simulink model "ADC2019"  (R2019b)
settings: Solver=VariableStepAuto  StartTime=0.0  StopTime=1  RelTol=1e-3
values from neighbouring files (symbols this model uses):
  Cf = minimum_cap    [SignalProcessing_SAR.m]    (also in simVariables.mat = 1.995e-15)
  clk_period = 1/clk_freq    [SignalProcessing_SAR.m]    (also in simVariables.mat = 5.92094282336e-05)
  comparator_high_offset = 8e-4    (= 0.0008)    [SignalProcessing_SAR.m]    (also in simVariables.mat)
  comparator_low_offset = 8e-4    (= 0.0008)    [SignalProcessing_SAR.m]    (also in simVariables.mat)
  comparator_noise_on = non_idealities_on    (= 1)    [SignalProcessing_SAR.m]    (also in simVariables.mat)
  comparator_noise_rms = 1*k*T* 2/3 / minimum_cap    [SignalProcessing_SAR.m]    (also in simVariables.mat = 1.35181292017e-06)
  comparator_offset_on = non_idealities_on    (= 1)    [SignalProcessing_SAR.m]    (also in simVariables.mat)
  k = 1.38064852e-23    [SignalProcessing_SAR.m]    (also in simVariables.mat)
  LNA_bandwidth = 30*input_BW    (= 7680)    [SignalProcessing_SAR.m]    (also in simVariables.mat)
  LNA_gain = 100    [SignalProcessing_SAR.m]    (also in simVariables.mat)
  LNA_input_referred_noise = min([LNA_input_referred_noise_1,LNA_input_referred_noise_2,LNA_input_referred_noise_3])    [SignalProcessing_SAR.m]    (also in simVariables.mat = 3.60843918244e-05)
  LNA_noise_on = non_idealities_on    (= 1)    [SignalProcessing_SAR.m]    (also in simVariables.mat)
  LNA_SR = I_LNA/(minimum_cap)    [SignalProcessing_SAR.m]    (also in simVariables.mat = 4429889.66082)
  number_of_bits = nb_bits    [SignalProcessing_SAR.m]    (also in simVariables.mat = 4)
  sample_time_jitter = 16e-12    (= 1.6e-11)    [SignalProcessing_SAR.m]    (also in simVariables.mat)
  sampling_gain = Cs/Cf    [SignalProcessing_SAR.m]    (also in simVariables.mat = 10)
  sampling_jitter_on = non_idealities_on    (= 1)    [SignalProcessing_SAR.m]    (also in simVariables.mat)
  switch_noise_on = non_idealities_on    (= 1)    [SignalProcessing_SAR.m]    (also in simVariables.mat)
  switching_noise = k*T/Cf    [SignalProcessing_SAR.m]    (also in simVariables.mat = 2.02771938025e-06)
  T = 293    [SignalProcessing_SAR.m]    (also in simVariables.mat)
  Vref = 2    [SignalProcessing_SAR.m]    (also in simVariables.mat)
undefined symbols (not defined in the file or in its folder): sim_number
libraries: dspsigops x2, spsFirstOrderFilterLib x1, simulink x1, simulink_extras x1, dspsrcs4 x1
settings Model: SnapshotInterval=1  Creator=mac  LastModifiedBy=mac
settings DataIOCC: SaveFormat=Structure  OutputOption=SpecifiedOutputTimes  OutputTimes=0:(clk_period*(number_of_bits+1)): length(ADC_input)*(number_of_bits+1)*clk_period
settings DebuggingCC: UnderSpecifiedDimensionMsg=warning

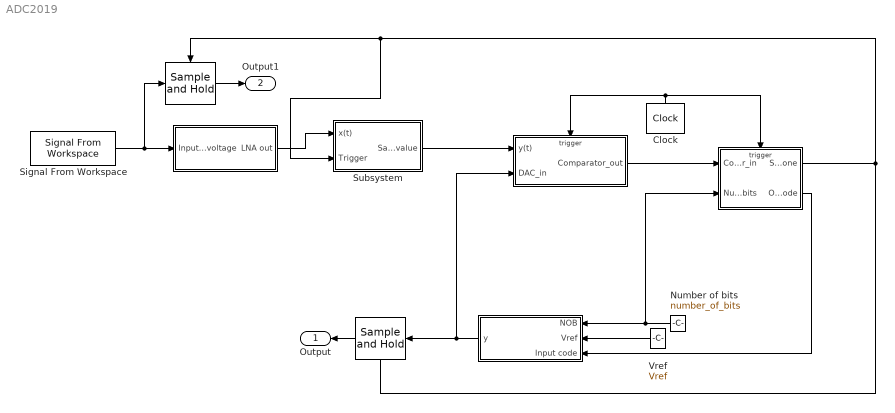
== system ADC2019 ==
  " " : Subsystem
      mask Display: text(.5, .5, 'LNA', 'horizontalAlignment', 'center', 'verticalAlignment', 'middle')
  "  " : Subsystem  TreatAsAtomicUnit=on
      mask Display: text(.5, .5, 'Comparator', 'horizontalAlignment', 'center', 'verticalAlignment', 'middle')
  "    " : Subsystem  TreatAsAtomicUnit=on
      mask Display: text(.5, .5, 'SAR', 'horizontalAlignment', 'center', 'verticalAlignment', 'middle')
  "       " : Subsystem  TreatAsAtomicUnit=on
      mask Display: text(.5, .5, 'DAC', 'horizontalAlignment', 'center', 'verticalAlignment', 'middle')
  "          " : dspsigops/Sample and Hold  trig=Rising edge  initCond=0  latchinput=off
  "           " : dspsigops/Sample and Hold  trig=Rising edge  initCond=0  latchinput=off
  Clock : simulink_extras/Flip Flops/Clock  period=clk_period
  Number of bits : Constant  Value=number_of_bits
  Signal From Workspace : dspsrcs4/Signal From Workspace  X=ADC_input  Ts=clk_period*(number_of_bits+1)  nsamps=1  OutputAfterFinalValue=Setting to zero  ignoreOrWarnInputAndFrameLengths=off  OutputFrames=off
  Subsystem : Subsystem
      mask Display: text(.5, .5, 'Sample & hold', 'horizontalAlignment', 'center', 'verticalAlignment', 'middle')
  Vref : Constant  Value=Vref
  Output : Outport
  Output1 : Outport  Port=2
  wires:
  Vref/1 -> "       "/2(Vref)
  "    "/2(Output_code) -> "       "/3(Input code)
  Clock/1 -> "    "/Trigger, "  "/Trigger
  "       "/1(y) -> "           "/1, "  "/2(DAC_in)
  "  "/1(Comparator_out) -> "    "/1(Comparator_in)
  "           "/1 -> Output/1
  " "/1(LNA out) -> Subsystem/1(x(t))
  Subsystem/1(Sampled value) -> "  "/1(y(t))
  Number of bits/1 -> "    "/2(Number of bits), "       "/1(NOB)
  "    "/1(SAR_done) -> "           "/Trigger, Subsystem/2(Trigger), "          "/Trigger
  Signal From Workspace/1 -> "          "/1, " "/1(Input voltage)
  "          "/1 -> Output1/1

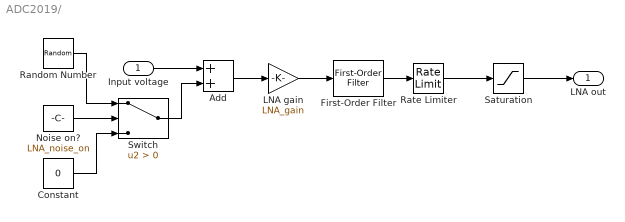
== system ADC2019/  ==
  Input voltage : Inport
  Add : Sum
  Constant : Constant  Value=0
  "First-Order Filter " : spsFirstOrderFilterLib/First-Order Filter  FilterType=Lowpass  Tc=1/(LNA_bandwidth*2*pi)  Ts=0  Initialize=on  Vac_Init=[0, 0, 60]  Vdc_Init=0  PlotResponse=off  FreqRange="[0,  200,  1]"
  LNA gain : Gain  Gain=LNA_gain
  Noise on? : Constant  Value=LNA_noise_on
  "Random Number " : RandomNumber  Variance=LNA_input_referred_noise^2  Seed=sim_number+100  SampleTime=clk_period*(number_of_bits+1)
  Rate Limiter : RateLimiter  RisingSlewLimit=LNA_SR  FallingSlewLimit=-LNA_SR  SampleTimeMode=inherited
  Saturation : Saturate  UpperLimit=Vref  LowerLimit=0
  Switch : Switch  Criteria=u2 > Threshold
  LNA out : Outport
  wires:
  Input voltage/1 -> Add/1
  Add/1 -> LNA gain/1
  Constant/1 -> Switch/3
  Noise on?/1 -> Switch/2
  Switch/1 -> Add/2
  "Random Number "/1 -> Switch/1
  "First-Order Filter "/1 -> Rate Limiter/1
  Rate Limiter/1 -> Saturation/1
  LNA gain/1 -> "First-Order Filter "/1
  Saturation/1 -> LNA out/1

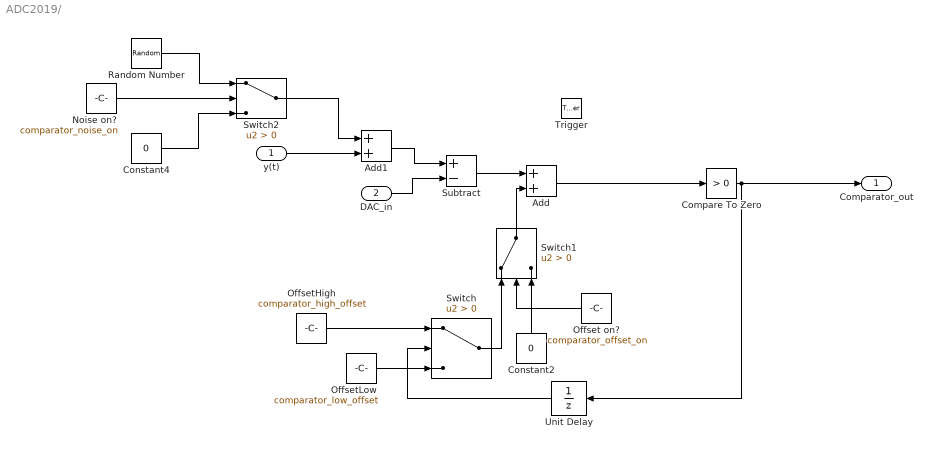
== system ADC2019/   ==
  y(t) : Inport
  DAC_in : Inport  Port=2
  Trigger : TriggerPort  VariantControl=Variant
  Add : Sum
  Add1 : Sum
  Compare To Zero : simulink/Logic and Bit Operations/Compare To Zero  relop=>  OutDataTypeStr=boolean
  Constant2 : Constant  Value=0
  Constant4 : Constant  Value=0
  Noise on? : Constant  Value=comparator_noise_on
  Offset on? : Constant  Value=comparator_offset_on
  OffsetHigh : Constant  Value=comparator_high_offset  VectorParams1D=off
  OffsetLow : Constant  Value=comparator_low_offset
  "Random Number " : RandomNumber  Variance=comparator_noise_rms^2  Seed=sim_number+420
  Subtract : Sum  Inputs=+-
  Switch : Switch  Criteria=u2 > Threshold
  Switch1 : Switch  Criteria=u2 > Threshold
  Switch2 : Switch  Criteria=u2 > Threshold
  Unit Delay : UnitDelay  SampleTime=-1  HasFrameUpgradeWarning=on
  Comparator_out : Outport
  wires:
  Switch/1 -> Switch1/1
  Subtract/1 -> Add/1
  OffsetHigh/1 -> Switch/1
  Constant2/1 -> Switch1/3
  Switch1/1 -> Add/2
  Offset on?/1 -> Switch1/2
  Unit Delay/1 -> Switch/2
  OffsetLow/1 -> Switch/3
  DAC_in/1 -> Subtract/2
  Add1/1 -> Subtract/1
  y(t)/1 -> Add1/2
  Switch2/1 -> Add1/1
  "Random Number "/1 -> Switch2/1
  Constant4/1 -> Switch2/3
  Noise on?/1 -> Switch2/2
  Add/1 -> Compare To Zero/1
  Compare To Zero/1 -> Unit Delay/1, Comparator_out/1

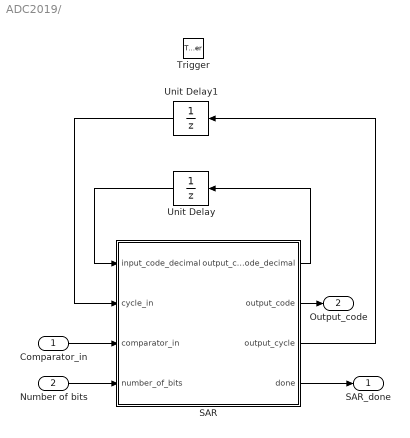
== system ADC2019/     ==
  Comparator_in : Inport  LatchByDelayingOutsideSignal=on
  Number of bits : Inport  Port=2
  Trigger : TriggerPort  VariantControl=Variant
  SAR : MATLAB Function  TreatAsAtomicUnit=on
  Unit Delay : UnitDelay  SampleTime=-1  HasFrameUpgradeWarning=on
  Unit Delay1 : UnitDelay  SampleTime=-1  HasFrameUpgradeWarning=on
  SAR_done : Outport
  Output_code : Outport  Port=2  InitialOutput=zeros(number_of_bits,1)
      settings: VarSizeSig=Yes
  wires:
  Number of bits/1 -> SAR/4(number_of_bits)
  Comparator_in/1 -> SAR/3(comparator_in)
  SAR/4(done) -> SAR_done/1
  SAR/3(output_cycle) -> Unit Delay1/1
  Unit Delay1/1 -> SAR/2(cycle_in)
  SAR/2(output_code) -> Output_code/1
  Unit Delay/1 -> SAR/1(input_code_decimal)
  SAR/1(output_code_decimal) -> Unit Delay/1

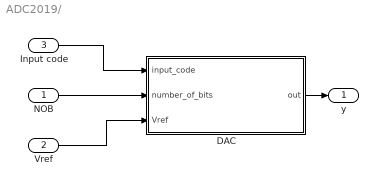
== system ADC2019/        ==
  NOB : Inport
  Vref : Inport  Port=2
  Input code : Inport  Port=3
  DAC : MATLAB Function  TreatAsAtomicUnit=on
  y : Outport
  wires:
  NOB/1 -> DAC/2(number_of_bits)
  Vref/1 -> DAC/3(Vref)
  DAC/1(out) -> y/1
  Input code/1 -> DAC/1(input_code)

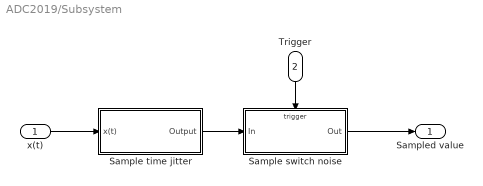
== system ADC2019/Subsystem ==
  x(t) : Inport
  Trigger : Inport  Port=2
  Sample switch noise : Subsystem  TreatAsAtomicUnit=on
  Sample time jitter : Subsystem
  Sampled value : Outport
  wires:
  x(t)/1 -> Sample time jitter/1(x(t))
  Trigger/1 -> Sample switch noise/Trigger
  Sample switch noise/1(Out) -> Sampled value/1
  Sample time jitter/1(Output) -> Sample switch noise/1(In)

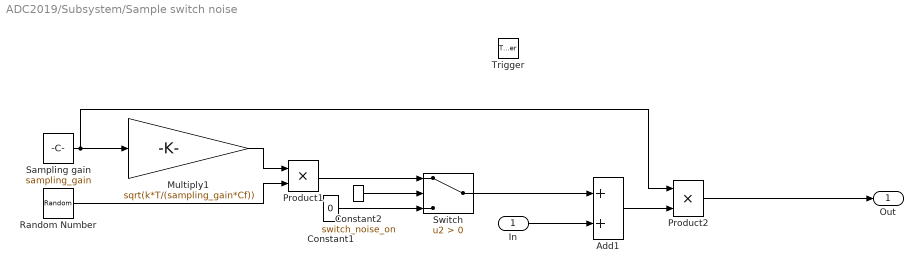
== system ADC2019/Subsystem/Sample switch noise ==
  In : Inport
  Trigger : TriggerPort  VariantControl=Variant
  Add1 : Sum
  Constant1 : Constant  Value=0
  Constant2 : Constant  Value=switch_noise_on
  Multiply1 : Gain  Gain=sqrt(k*T/(sampling_gain*Cf))  OutDataTypeStr=Inherit: Same as input
  Product1 : Product
  Product2 : Product
  "Random Number  " : RandomNumber  Variance=switching_noise  Seed=sim_number+69
  Sampling gain : Constant  Value=sampling_gain
  Switch : Switch  Criteria=u2 > Threshold
  Out : Outport
  wires:
  Product2/1 -> Out/1
  Multiply1/1 -> Product1/1
  Add1/1 -> Product2/2
  Sampling gain/1 -> Product2/1, Multiply1/1
  Constant2/1 -> Switch/2
  Constant1/1 -> Switch/3
  Product1/1 -> Switch/1
  "Random Number  "/1 -> Product1/2
  Switch/1 -> Add1/1
  In/1 -> Add1/2

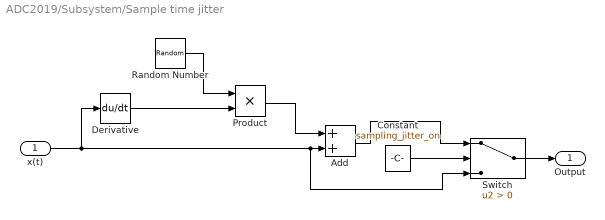
== system ADC2019/Subsystem/Sample time jitter ==
  x(t) : Inport
  Add : Sum
  Constant : Constant  Value=sampling_jitter_on
  Derivative : Derivative
  Product : Product
  "Random Number " : RandomNumber  Variance=sample_time_jitter^2  Seed=sim_number-1  SampleTime=clk_period*(number_of_bits+1)
  Switch : Switch  Criteria=u2 > Threshold
  Output : Outport
  wires:
  Switch/1 -> Output/1
  Add/1 -> Switch/1
  Constant/1 -> Switch/2
  x(t)/1 -> Derivative/1, Add/2, Switch/3
  Product/1 -> Add/1
  Derivative/1 -> Product/2
  "Random Number "/1 -> Product/1

== matlab function ADC2019/       /DAC ==
  data: input_code input size=number_of_bits; out output double size=1; number_of_bits input; Vref input
function out = fcn(input_code, number_of_bits, Vref)
out = Vref/(2^number_of_bits)*(bi2de(input_code.', 'left-msb'));
end

== matlab function ADC2019/    /SAR ==
  data: output_code_decimal output size=1; input_code_decimal input; output_code output size=number_of_bits; cycle_in input; comparator_in input; number_of_bits input; output_cycle output size=1; done output
function [output_code_decimal, output_code, output_cycle, done] = fcn(input_code_decimal, cycle_in, comparator_in, number_of_bits)

    input_code = de2bi(input_code_decimal, 'left-msb');
    output_code = [zeros(number_of_bits-size(input_code.',1),1); input_code.'];


    if (cycle_in == number_of_bits)
        done = 1;
        output_code(number_of_bits,1) = comparator_in;
        output_cycle = 0;

    elseif (cycle_in == 0)

        output_code = zeros(number_of_bits,1);
        output_code(1, 1) = 1;
        done=0;
        output_cycle = 1;

    else

        if (comparator_in == 0)
            output_code(cycle_in,1) = 0;
        end

        output_code(cycle_in+1,1)=1;
        output_cycle = cycle_in+1;
        done=0;
    end
    output_code_decimal_temp = bi2de(output_code.', 'left-msb');
    output_code_decimal = output_code_decimal_temp(1,1);
end
